simulink model "chap11_10sim"  (Simulink 7.7)
settings: Solver=ode45  StartTime=0.0  StopTime=10  FixedStep=0.001  RelTol=1e-3
settings Model: Creator=ljk  LastModifiedBy=ljk  ExtModeTrigMode=oneshot  ExtModeArmWhenConnect=off
settings DataIOCC: LimitDataPoints=off  SignalLoggingName=sigsOut
settings OptimizationCC: BooleanDataType=off
settings DebuggingCC: SaveWithParameterizedLinksMsg=none  SignalResolutionControl=TryResolveAllWithWarning  SolverPrmCheckMsg=none  MultiTaskDSMMsg=warning  MultiTaskCondExecSysMsg=none  StrictBusMsg=None
settings HardwareCC: TargetIntDivRoundTo=Zero  TargetEndianess=LittleEndian  TargetHWDeviceType=MATLAB Host  ProdEqTarget=off
settings RTWCC: IncludeERTFirstTime=on
settings CodeAppCC: CustomSymbolStrType=$N$R$M_T

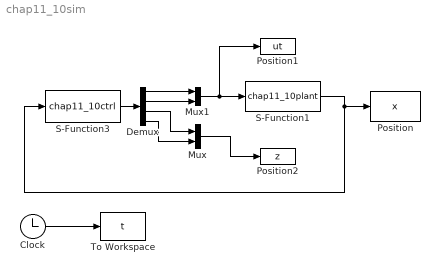
== system chap11_10sim ==
  Clock : Clock
      settings: Decimation=10
  Demux : Demux
  Mux : Mux  Inputs=2
  Mux1 : Mux  Inputs=2
  Position : ToWorkspace  VariableName=x  SampleTime=-1  SaveFormat=Array
  Position1 : ToWorkspace  VariableName=ut  SampleTime=-1  SaveFormat=Array
  Position2 : ToWorkspace  VariableName=z  SampleTime=-1  SaveFormat=Array
  S-Function1 : S-Function  FunctionName=chap11_10plant  EnableBusSupport=off
  S-Function3 : S-Function  FunctionName=chap11_10ctrl  EnableBusSupport=off
  To Workspace : ToWorkspace  VariableName=t  SampleTime=-1  SaveFormat=Array
  wires:
  Clock/1 -> To Workspace/1
  S-Function1/1 -> S-Function3/1, Position/1
  S-Function3/1 -> Demux/1
  Demux/3 -> Mux/1
  Demux/4 -> Mux/2
  Demux/1 -> Mux1/1
  Demux/2 -> Mux1/2
  Mux1/1 -> Position1/1, S-Function1/1
  Mux/1 -> Position2/1
